simulink model "motor_ctr"  (R2020b)
settings: Solver=VariableStepAuto  StartTime=0.0  StopTime=10.0  RelTol=1e-3
settings Model: DataDictionary=dic_motor.sldd  OrderedModelArguments=off  Creator=com  LastModifiedBy=com
settings SolverCC: MaxConsecutiveMinStep=3
settings DebuggingCC: AlgebraicLoopMsg=none

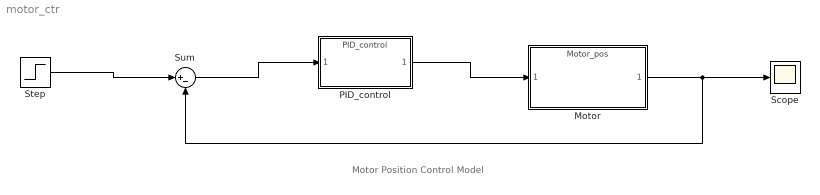
== system motor_ctr ==
  note: Motor Position Control Model
  Motor : ModelReference  ModelNameDialog=Motor_pos  ModelReferenceVersion=1.6
  PID_control : ModelReference  ModelNameDialog=PID_control  ModelReferenceVersion=1.6
  Scope : Scope
  Step : Step  After=500  SampleTime=0
  Sum : Sum  Inputs=|+-
  wires:
  Motor/1 -> Sum/2, Scope/1
  Step/1 -> Sum/1
  Sum/1 -> PID_control/1
  PID_control/1 -> Motor/1
